simulink library "INP_DRVR_ManOver"  (R2024b)
settings: Solver=VariableStepAuto  StartTime=0.0  StopTime=10.0  RelTol=1e-3
undefined symbols (not defined in the file): INP_DRVR_p_AngRatStWhlLoLim_radps, INP_DRVR_p_AngRatStWhlUpLim_radps, INP_DRVR_p_AngStWhlLoLim_rad, INP_DRVR_p_AngStWhlUpLim_rad, INP_DRVR_p_PosRatThrLoLim_p100ps, INP_DRVR_p_PosRatThrMan_p100ps, INP_DRVR_p_PosRatThrUpLim_p100ps, INP_DRVR_p_PosThrLoLim_p100, INP_DRVR_p_PosThrMan_p100, INP_DRVR_p_PosThrUpLim_p100, INP_DRVR_p_SwtAngRatStWhlMan_na, INP_DRVR_p_SwtAngStWhlMan_na, INP_DRVR_p_SwtPosRatThrMan_na, INP_DRVR_p_SwtPosThrMan_na, INP_DRVR_s_AngRatStWhlMan_radps, INP_DRVR_s_AngStWhlMan_rad
libraries: simulink x4
settings Model: Creator=blatak  LastModifiedBy=jmbsp

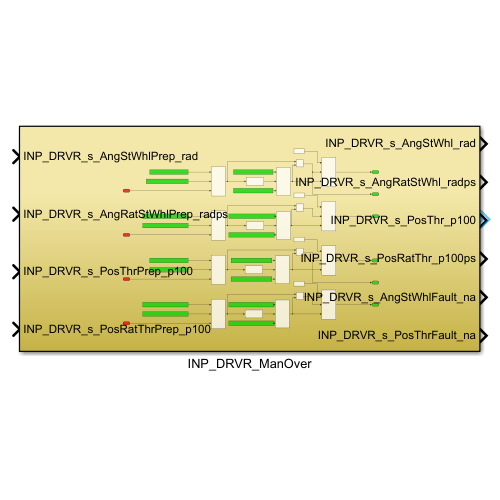
[thumbnail: Simulink's stored preview of the top-level diagram]
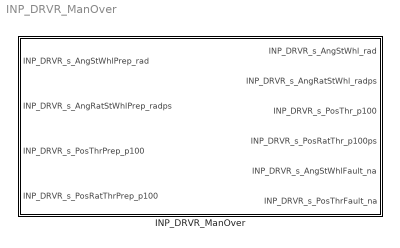
== system INP_DRVR_ManOver ==
  INP_DRVR_ManOver : Subsystem

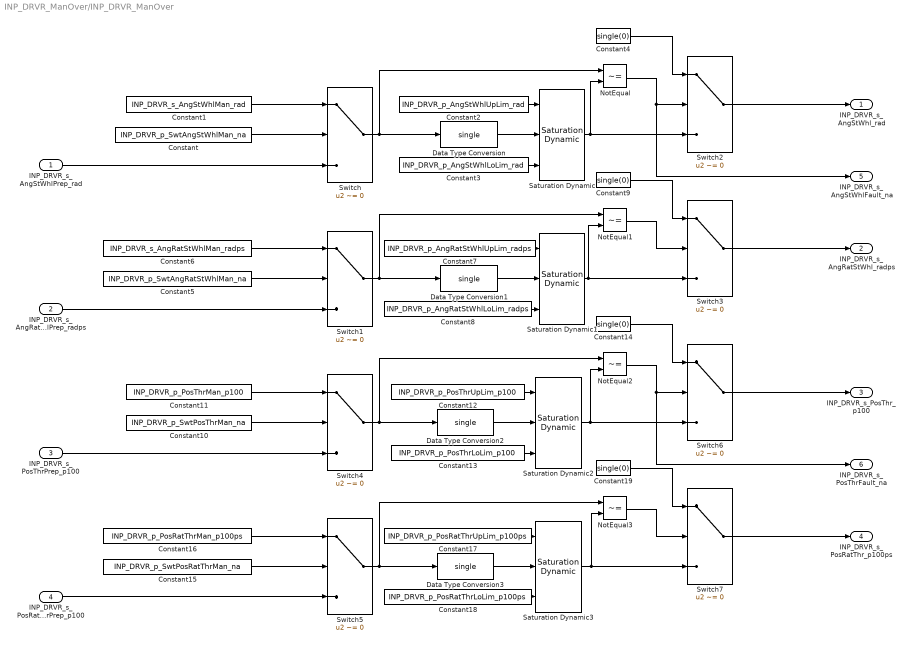
== system INP_DRVR_ManOver/INP_DRVR_ManOver ==
  INP_DRVR_s_AngStWhlPrep_rad : Inport
  INP_DRVR_s_AngRatStWhlPrep_radps : Inport  Port=2
  INP_DRVR_s_PosThrPrep_p100 : Inport  Port=3
  INP_DRVR_s_PosRatThrPrep_p100 : Inport  Port=4
  Constant : Constant  Description=|  Value=INP_DRVR_p_SwtAngStWhlMan_na
      | Switch for manual override of the longitudinal acceleration value, if 1 instead the measured 
      | value the INP_IMU_p_ALgtVehMan_mps2 is used
  Constant1 : Constant  Description=|  Value=INP_DRVR_s_AngStWhlMan_rad
      | Value for longitudinal acceleration, which is used if the INP_IMU_p_SwtAXxxVehMan_na
      | is set to 1 instead of the measured value
  Constant10 : Constant  Description=|  Value=INP_DRVR_p_SwtPosThrMan_na
      | Switch for manual override of the longitudinal acceleration value, if 1 instead the measured 
      | value the INP_IMU_p_ALgtVehMan_mps2 is used
  Constant11 : Constant  Description=|  Value=INP_DRVR_p_PosThrMan_p100
      | Value for longitudinal acceleration, which is used if the INP_IMU_p_SwtAXxxVehMan_na
      | is set to 1 instead of the measured value
  Constant12 : Constant  Description=Upper saturation limit for longitudinal acceleration  Value=INP_DRVR_p_PosThrUpLim_p100
  Constant13 : Constant  Description=Lower saturation limit for longitudinal acceleration  Value=INP_DRVR_p_PosThrLoLim_p100
  Constant{4,9,14,19} (4 alike) : Constant  Value=single(0)
  Constant15 : Constant  Description=|  Value=INP_DRVR_p_SwtPosRatThrMan_na
      | Switch for manual override of the longitudinal acceleration value, if 1 instead the measured 
      | value the INP_IMU_p_ALgtVehMan_mps2 is used
  Constant16 : Constant  Description=|  Value=INP_DRVR_p_PosRatThrMan_p100ps
      | Value for longitudinal acceleration, which is used if the INP_IMU_p_SwtAXxxVehMan_na
      | is set to 1 instead of the measured value
  Constant17 : Constant  Description=Upper saturation limit for longitudinal acceleration  Value=INP_DRVR_p_PosRatThrUpLim_p100ps
  Constant18 : Constant  Description=Lower saturation limit for longitudinal acceleration  Value=INP_DRVR_p_PosRatThrLoLim_p100ps
  Constant2 : Constant  Description=Upper saturation limit for longitudinal acceleration  Value=INP_DRVR_p_AngStWhlUpLim_rad
  Constant3 : Constant  Description=Lower saturation limit for longitudinal acceleration  Value=INP_DRVR_p_AngStWhlLoLim_rad
  Constant5 : Constant  Description=|  Value=INP_DRVR_p_SwtAngRatStWhlMan_na
      | Switch for manual override of the longitudinal acceleration value, if 1 instead the measured 
      | value the INP_IMU_p_ALgtVehMan_mps2 is used
  Constant6 : Constant  Description=|  Value=INP_DRVR_s_AngRatStWhlMan_radps
      | Value for longitudinal acceleration, which is used if the INP_IMU_p_SwtAXxxVehMan_na
      | is set to 1 instead of the measured value
  Constant7 : Constant  Description=Upper saturation limit for longitudinal acceleration  Value=INP_DRVR_p_AngRatStWhlUpLim_radps
  Constant8 : Constant  Description=Lower saturation limit for longitudinal acceleration  Value=INP_DRVR_p_AngRatStWhlLoLim_radps
  Data Type Conversion{,1..3} (4 alike) : DataTypeConversion  OutDataTypeStr=single  SaturateOnIntegerOverflow=off  RndMeth=Floor
  NotEqual{,1..3} (4 alike) : RelationalOperator  Operator=~=  OutDataTypeStr=boolean  RndMeth=Simplest  InputSameDT=off
  Saturation Dynamic{,1..3} (4 alike) : simulink/Discontinuities/Saturation Dynamic  OutMin=[]  OutMax=[]  OutDataTypeStr=Inherit: Same as second input  OutDataType=fixdt(1, 16)  OutScaling=2^-10  DoSatur=off
  Switch{,1..7} (8 alike) : Switch  Criteria=u2 ~= 0  SaturateOnIntegerOverflow=off  InputSameDT=off
  INP_DRVR_s_AngStWhl_rad : Outport
  INP_DRVR_s_AngRatStWhl_radps : Outport  Port=2
  INP_DRVR_s_PosThr_p100 : Outport  Port=3
  INP_DRVR_s_PosRatThr_p100ps : Outport  Port=4
  INP_DRVR_s_AngStWhlFault_na : Outport  Port=5
  INP_DRVR_s_PosThrFault_na : Outport  Port=6
  wires:
  Switch3/1 -> INP_DRVR_s_AngRatStWhl_radps/1
  Constant15/1 -> Switch5/2
  Constant12/1 -> Saturation Dynamic2/1
  Switch4/1 -> Data Type Conversion2/1, NotEqual2/1
  Constant11/1 -> Switch4/1
  Constant13/1 -> Saturation Dynamic2/3
  Constant7/1 -> Saturation Dynamic1/1
  Data Type Conversion/1 -> Saturation Dynamic/2
  Constant9/1 -> Switch3/1
  Saturation Dynamic/1 -> NotEqual/2, Switch2/3
  Data Type Conversion3/1 -> Saturation Dynamic3/2
  Saturation Dynamic3/1 -> NotEqual3/2, Switch7/3
  Switch1/1 -> Data Type Conversion1/1, NotEqual1/1
  NotEqual2/1 -> INP_DRVR_s_PosThrFault_na/1, Switch6/2
  Constant19/1 -> Switch7/1
  INP_DRVR_s_AngStWhlPrep_rad/1 -> Switch/3
  Constant17/1 -> Saturation Dynamic3/1
  Switch/1 -> Data Type Conversion/1, NotEqual/1
  INP_DRVR_s_PosRatThrPrep_p100/1 -> Switch5/3
  Saturation Dynamic1/1 -> NotEqual1/2, Switch3/3
  INP_DRVR_s_PosThrPrep_p100/1 -> Switch4/3
  Constant3/1 -> Saturation Dynamic/3
  Constant6/1 -> Switch1/1
  Constant18/1 -> Saturation Dynamic3/3
  Saturation Dynamic2/1 -> NotEqual2/2, Switch6/3
  Constant8/1 -> Saturation Dynamic1/3
  Constant4/1 -> Switch2/1
  Switch6/1 -> INP_DRVR_s_PosThr_p100/1
  Switch5/1 -> Data Type Conversion3/1, NotEqual3/1
  NotEqual3/1 -> Switch7/2
  Switch2/1 -> INP_DRVR_s_AngStWhl_rad/1
  Constant16/1 -> Switch5/1
  Data Type Conversion2/1 -> Saturation Dynamic2/2
  Constant10/1 -> Switch4/2
  NotEqual/1 -> INP_DRVR_s_AngStWhlFault_na/1, Switch2/2
  Constant14/1 -> Switch6/1
  NotEqual1/1 -> Switch3/2
  Switch7/1 -> INP_DRVR_s_PosRatThr_p100ps/1
  Constant1/1 -> Switch/1
  Constant5/1 -> Switch1/2
  INP_DRVR_s_AngRatStWhlPrep_radps/1 -> Switch1/3
  Constant2/1 -> Saturation Dynamic/1
  Data Type Conversion1/1 -> Saturation Dynamic1/2
  Constant/1 -> Switch/2
